simulink model "trikompar"  (Simulink 8.0)
settings: Solver=ode45  StartTime=0.0  StopTime=100  RelTol=1e-3
settings Model: Creator=polacmi1  LastModifiedBy=Jarda
settings DataIOCC: SignalLoggingSaveFormat=ModelDataLogs
settings DebuggingCC: FcnCallInpInsideContextMsg=EnableAllAsWarning

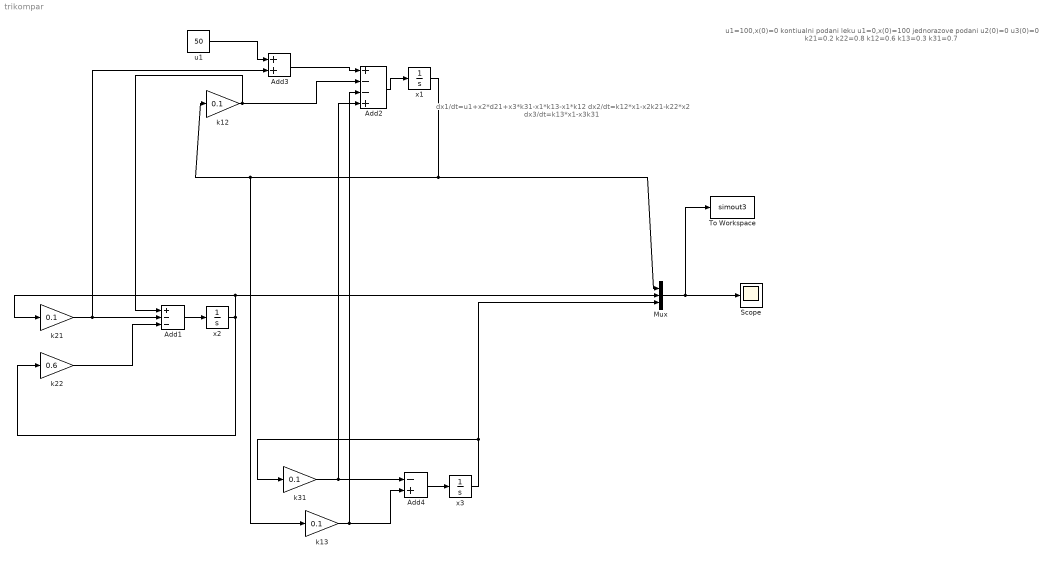
== system trikompar ==
  note: u1=100,x(0)=0 kontiualni podani leku
      | u1=0,x(0)=100 jednorazove podani
      | u2(0)=0
      | u3(0)=0
      | k21=0.2
      | k22=0.8
      | k12=0.6
      | k13=0.3
      | k31=0.7
  note: dx1/dt=u1+x2*d21+x3*k31-x1*k13-x1*k12
      |
      | dx2/dt=k12*x1-x2k21-k22*x2
      |
      | dx3/dt=k13*x1-x3k31
  Add1 : Sum  Inputs=+--
  Add2 : Sum  Inputs=+--+
  Add3 : Sum
  Add4 : Sum  Inputs=-+
  Mux : Mux  Inputs=3
  Scope : Scope
  To Workspace : ToWorkspace  VariableName=simout3  SampleTime=-1  SaveFormat=Timeseries
  k{12..13,21,31} (4 alike) : Gain  Gain=0.1
  k22 : Gain  Gain=0.6
  u1 : Constant  Value=50
  x1 : Integrator
  x2 : Integrator
  x3 : Integrator
  wires:
  x1/1 -> k12/1, k13/1, Mux/1
  x2/1 -> k22/1, k21/1, Mux/2
  Add1/1 -> x2/1
  Add2/1 -> x1/1
  k12/1 -> Add2/2, Add1/1
  u1/1 -> Add3/1
  k21/1 -> Add1/2, Add3/2
  Add3/1 -> Add2/1
  Mux/1 -> To Workspace/1, Scope/1
  k22/1 -> Add1/3
  x3/1 -> k31/1, Mux/3
  Add4/1 -> x3/1
  k31/1 -> Add2/4, Add4/1
  k13/1 -> Add4/2, Add2/3
